simulink model "ep10_23"  (R2018a)
settings: Solver=VariableStepAuto  StartTime=0.0  StopTime=10.0  RelTol=1e-3
libraries: simulink x1
settings Model: Creator=zheny  LastModifiedBy=zheny

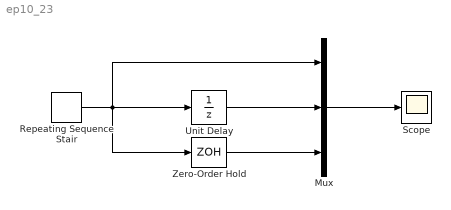
== system ep10_23 ==
  Mux : Mux  Inputs=3
  Repeating Sequence Stair : simulink/Sources/Repeating Sequence Stair  OutValues=[1:8].'  tsamp=1  OutMin=[]  OutMax=[]  OutDataTypeStr=double  OutputDataTypeScalingMode=double  OutDataType=fixdt(0,8)  ConRadixGroup=Best Precision: Vector-wise  OutScaling=2^-12
  Scope : Scope
  Unit Delay : UnitDelay  SampleTime=-1
  Zero-Order Hold : ZeroOrderHold  SampleTime=-1
  wires:
  Zero-Order Hold/1 -> Mux/3
  Unit Delay/1 -> Mux/2
  Repeating Sequence Stair/1 -> Mux/1, Zero-Order Hold/1, Unit Delay/1
  Mux/1 -> Scope/1
